simulink model "case6"  (R2024b)
settings: Solver=FixedStepAuto  StartTime=0  StopTime=1  FixedStep=1e-7  RelTol=1e-3
values from neighbouring files (symbols this model uses):
  SG_D_1_D = 0.01056    [IEEE9_case_parameters.m]    (also in case1_parameters.m; case2_parameters.m; case3_parameters.m; case4_parameters.m)
  SG_D_1_EnableSaturation = 0    [IEEE9_case_parameters.m]    (also in case1_parameters.m; case2_parameters.m; case3_parameters.m; case4_parameters.m)
  SG_D_1_f0 = 60    [IEEE9_case_parameters.m]    (also in case1_parameters.m; case2_parameters.m; case3_parameters.m; case4_parameters.m)
  SG_D_1_H = 7.5    [IEEE9_case_parameters.m]    (also in case1_parameters.m; case2_parameters.m; case3_parameters.m; case4_parameters.m)
  SG_D_1_K_A = 20    [IEEE9_case_parameters.m]    (also in case1_parameters.m; case2_parameters.m; case3_parameters.m; case4_parameters.m)
  SG_D_1_K_E = 1.000000e+1    (= 10)    [IEEE9_case_parameters.m]    (also in case1_parameters.m; case2_parameters.m; case3_parameters.m; case4_parameters.m)
  SG_D_1_K_F = 2.363    [IEEE9_case_parameters.m]    (also in case1_parameters.m; case2_parameters.m; case3_parameters.m; case4_parameters.m)
  SG_D_1_K_s = 0.5    [IEEE9_case_parameters.m]    (also in case1_parameters.m = 5; case2_parameters.m = 5; case3_parameters.m = 5; case4_parameters.m = 5)
  SG_D_1_R_a = 0.001088    [IEEE9_case_parameters.m]    (also in case1_parameters.m; case2_parameters.m; case3_parameters.m; case4_parameters.m)
  SG_D_1_S_A = 1    [IEEE9_case_parameters.m]    (also in case1_parameters.m; case2_parameters.m; case3_parameters.m; case4_parameters.m)
  SG_D_1_S_B = 0.103    [IEEE9_case_parameters.m]    (also in case1_parameters.m; case2_parameters.m; case3_parameters.m; case4_parameters.m)
  SG_D_1_S_N = 10.659857    [IEEE9_case_parameters.m]    (also in case1_parameters.m; case2_parameters.m; case3_parameters.m; case4_parameters.m)
  SG_D_1_SpeedPara = 200    [IEEE9_case_parameters.m]    (also in case1_parameters.m; case2_parameters.m; case3_parameters.m; case4_parameters.m)
  SG_D_1_T_0 = 0.720173    [IEEE9_case_parameters.m]    (also in case1_parameters.m = 0.755522; case2_parameters.m = 0.808931; case3_parameters.m = 0.869402; case4_parameters.m = 0.729316)
  SG_D_1_T_1 = 0.3    [IEEE9_case_parameters.m]    (also in case1_parameters.m; case2_parameters.m; case3_parameters.m; case4_parameters.m)
  SG_D_1_T_2 = 0.05    [IEEE9_case_parameters.m]    (also in case1_parameters.m; case2_parameters.m; case3_parameters.m; case4_parameters.m)
  SG_D_1_T_3 = 0.02    [IEEE9_case_parameters.m]    (also in case1_parameters.m; case2_parameters.m; case3_parameters.m; case4_parameters.m)
  SG_D_1_T_4 = 0.005    [IEEE9_case_parameters.m]    (also in case1_parameters.m; case2_parameters.m; case3_parameters.m; case4_parameters.m)
  SG_D_1_T_A = 0.02    [IEEE9_case_parameters.m]    (also in case1_parameters.m; case2_parameters.m; case3_parameters.m; case4_parameters.m)
  SG_D_1_T_dd = 8.000000e+0    (= 8)    [IEEE9_case_parameters.m]    (also in case1_parameters.m; case2_parameters.m; case3_parameters.m; case4_parameters.m)
  SG_D_1_T_ddd = 0.04    [IEEE9_case_parameters.m]    (also in case1_parameters.m; case2_parameters.m; case3_parameters.m; case4_parameters.m)
  SG_D_1_T_E = 0.314    [IEEE9_case_parameters.m]    (also in case1_parameters.m; case2_parameters.m; case3_parameters.m; case4_parameters.m)
  SG_D_1_T_F = 0.35    [IEEE9_case_parameters.m]    (also in case1_parameters.m; case2_parameters.m; case3_parameters.m; case4_parameters.m)
  SG_D_1_T_qd = 0.8    [IEEE9_case_parameters.m]    (also in case1_parameters.m; case2_parameters.m; case3_parameters.m; case4_parameters.m)
  SG_D_1_T_qdd = 0.02    [IEEE9_case_parameters.m]    (also in case1_parameters.m; case2_parameters.m; case3_parameters.m; case4_parameters.m)
  SG_D_1_T_speed = 0.1    [IEEE9_case_parameters.m]    (also in case1_parameters.m = 200; case2_parameters.m = 200; case3_parameters.m = 200; case4_parameters.m = 200)
  SG_D_1_T_w = 0.5    [IEEE9_case_parameters.m]    (also in case1_parameters.m; case2_parameters.m; case3_parameters.m; case4_parameters.m)
  SG_D_1_V_ref = 1.990276    [IEEE9_case_parameters.m]    (also in case1_parameters.m = 2.042296; case2_parameters.m = 2.051388; case3_parameters.m = 2.089584; case4_parameters.m = 2.01845)
  SG_D_1_w_ref = 376.991118    [IEEE9_case_parameters.m]    (also in case1_parameters.m; case2_parameters.m; case3_parameters.m; case4_parameters.m)
  SG_D_1_wb = 6.000000e+1    (= 60)    [IEEE9_case_parameters.m]    (also in case1_parameters.m; case2_parameters.m; case3_parameters.m; case4_parameters.m)
  SG_D_1_x_d = 1.9    [IEEE9_case_parameters.m]    (also in case1_parameters.m; case2_parameters.m; case3_parameters.m; case4_parameters.m)
  SG_D_1_x_dd = 0.302    [IEEE9_case_parameters.m]    (also in case1_parameters.m; case2_parameters.m; case3_parameters.m; case4_parameters.m)
  SG_D_1_x_ddd = 0.204    [IEEE9_case_parameters.m]    (also in case1_parameters.m; case2_parameters.m; case3_parameters.m; case4_parameters.m)
  SG_D_1_x_l = 0.05    [IEEE9_case_parameters.m]    (also in case1_parameters.m; case2_parameters.m; case3_parameters.m; case4_parameters.m)
  SG_D_1_x_q = 1.3    [IEEE9_case_parameters.m]    (also in case1_parameters.m; case2_parameters.m; case3_parameters.m; case4_parameters.m)
  SG_D_1_x_qd = 0.5    [IEEE9_case_parameters.m]    (also in case1_parameters.m; case2_parameters.m; case3_parameters.m; case4_parameters.m)
  SG_D_1_x_qdd = 0.3    [IEEE9_case_parameters.m]    (also in case1_parameters.m; case2_parameters.m; case3_parameters.m; case4_parameters.m)
  SG_D_2_D = 0.02    [IEEE9_case_parameters.m]    (also in case1_parameters.m; case2_parameters.m; case3_parameters.m; case4_parameters.m)
  SG_D_2_EnableSaturation = 0    [IEEE9_case_parameters.m]    (also in case1_parameters.m; case2_parameters.m; case3_parameters.m; case4_parameters.m)
  SG_D_2_f0 = 60    [IEEE9_case_parameters.m]    (also in case1_parameters.m; case2_parameters.m; case3_parameters.m; case4_parameters.m)
  SG_D_2_H = 8.000000e+0    (= 8)    [IEEE9_case_parameters.m]    (also in case1_parameters.m; case2_parameters.m; case3_parameters.m; case4_parameters.m)
  SG_D_2_K_A = 20    [IEEE9_case_parameters.m]    (also in case1_parameters.m; case2_parameters.m; case3_parameters.m; case4_parameters.m)
  SG_D_2_K_E = 1.000000e+1    (= 10)    [IEEE9_case_parameters.m]    (also in case1_parameters.m; case2_parameters.m; case3_parameters.m; case4_parameters.m)
  SG_D_2_K_F = 2.363    [IEEE9_case_parameters.m]    (also in case1_parameters.m; case2_parameters.m; case3_parameters.m; case4_parameters.m)
  SG_D_2_K_s = 0.5    [IEEE9_case_parameters.m]    (also in case1_parameters.m = 4; case2_parameters.m = 4; case3_parameters.m = 4; case4_parameters.m = 4)
  SG_D_2_R_a = 0.001088    [IEEE9_case_parameters.m]    (also in case1_parameters.m; case2_parameters.m; case3_parameters.m; case4_parameters.m)
  SG_D_2_S_A = 1    [IEEE9_case_parameters.m]    (also in case1_parameters.m; case2_parameters.m; case3_parameters.m; case4_parameters.m)
  SG_D_2_S_B = 0.103    [IEEE9_case_parameters.m]    (also in case1_parameters.m; case2_parameters.m; case3_parameters.m; case4_parameters.m)
  SG_D_2_S_N = 10.659857    [IEEE9_case_parameters.m]    (also in case1_parameters.m; case2_parameters.m; case3_parameters.m; case4_parameters.m)
  SG_D_2_SpeedPara = 200    [IEEE9_case_parameters.m]    (also in case1_parameters.m; case2_parameters.m; case3_parameters.m; case4_parameters.m)
  SG_D_2_T_0 = 1.632913    [IEEE9_case_parameters.m]    (also in case1_parameters.m = 1.632925; case2_parameters.m = 1.632915; case3_parameters.m = 1.632914; case4_parameters.m = 1.632927)
  SG_D_2_T_1 = 0.2    [IEEE9_case_parameters.m]    (also in case1_parameters.m; case2_parameters.m; case3_parameters.m; case4_parameters.m)
  SG_D_2_T_2 = 0.05    [IEEE9_case_parameters.m]    (also in case1_parameters.m; case2_parameters.m; case3_parameters.m; case4_parameters.m)
  SG_D_2_T_3 = 0.02    [IEEE9_case_parameters.m]    (also in case1_parameters.m; case2_parameters.m; case3_parameters.m; case4_parameters.m)
  SG_D_2_T_4 = 0.005    [IEEE9_case_parameters.m]    (also in case1_parameters.m; case2_parameters.m; case3_parameters.m; case4_parameters.m)
  SG_D_2_T_A = 0.02    [IEEE9_case_parameters.m]    (also in case1_parameters.m; case2_parameters.m; case3_parameters.m; case4_parameters.m)
  SG_D_2_T_dd = 7.9    [IEEE9_case_parameters.m]    (also in case1_parameters.m; case2_parameters.m; case3_parameters.m; case4_parameters.m)
  SG_D_2_T_ddd = 0.04    [IEEE9_case_parameters.m]    (also in case1_parameters.m; case2_parameters.m; case3_parameters.m; case4_parameters.m)
  SG_D_2_T_E = 0.314    [IEEE9_case_parameters.m]    (also in case1_parameters.m; case2_parameters.m; case3_parameters.m; case4_parameters.m)
  SG_D_2_T_F = 0.35    [IEEE9_case_parameters.m]    (also in case1_parameters.m; case2_parameters.m; case3_parameters.m; case4_parameters.m)
  SG_D_2_T_qd = 0.8    [IEEE9_case_parameters.m]    (also in case1_parameters.m; case2_parameters.m; case3_parameters.m; case4_parameters.m)
  SG_D_2_T_qdd = 0.015    [IEEE9_case_parameters.m]    (also in case1_parameters.m; case2_parameters.m; case3_parameters.m; case4_parameters.m)
  SG_D_2_T_speed = 0.1    [IEEE9_case_parameters.m]    (also in case1_parameters.m = 150; case2_parameters.m = 150; case3_parameters.m = 150; case4_parameters.m = 150)
  SG_D_2_T_w = 0.35    [IEEE9_case_parameters.m]    (also in case1_parameters.m; case2_parameters.m; case3_parameters.m; case4_parameters.m)
  SG_D_2_V_ref = 2.58547    [IEEE9_case_parameters.m]    (also in case1_parameters.m = 2.597896; case2_parameters.m = 2.587136; case3_parameters.m = 2.586042; case4_parameters.m = 2.599679)
  SG_D_2_w_ref = 376.991118    [IEEE9_case_parameters.m]    (also in case1_parameters.m; case2_parameters.m; case3_parameters.m; case4_parameters.m)
  SG_D_2_wb = 6.000000e+1    (= 60)    [IEEE9_case_parameters.m]    (also in case1_parameters.m; case2_parameters.m; case3_parameters.m; case4_parameters.m)
  SG_D_2_x_d = 1.8    [IEEE9_case_parameters.m]    (also in case1_parameters.m; case2_parameters.m; case3_parameters.m; case4_parameters.m)
  SG_D_2_x_dd = 0.302    [IEEE9_case_parameters.m]    (also in case1_parameters.m; case2_parameters.m; case3_parameters.m; case4_parameters.m)
  SG_D_2_x_ddd = 0.204    [IEEE9_case_parameters.m]    (also in case1_parameters.m; case2_parameters.m; case3_parameters.m; case4_parameters.m)
  SG_D_2_x_l = 0.05    [IEEE9_case_parameters.m]    (also in case1_parameters.m; case2_parameters.m; case3_parameters.m; case4_parameters.m)
  SG_D_2_x_q = 1.25    [IEEE9_case_parameters.m]    (also in case1_parameters.m; case2_parameters.m; case3_parameters.m; case4_parameters.m)
  SG_D_2_x_qd = 0.5    [IEEE9_case_parameters.m]    (also in case1_parameters.m; case2_parameters.m; case3_parameters.m; case4_parameters.m)
  SG_D_2_x_qdd = 0.3    [IEEE9_case_parameters.m]    (also in case1_parameters.m; case2_parameters.m; case3_parameters.m; case4_parameters.m)
  SG_D_3_D = 0.02    [IEEE9_case_parameters.m]    (also in case1_parameters.m; case2_parameters.m; case3_parameters.m; case4_parameters.m)
  SG_D_3_EnableSaturation = 0    [IEEE9_case_parameters.m]    (also in case1_parameters.m; case2_parameters.m; case3_parameters.m; case4_parameters.m)
  SG_D_3_f0 = 60    [IEEE9_case_parameters.m]    (also in case1_parameters.m; case2_parameters.m; case3_parameters.m; case4_parameters.m)
  SG_D_3_H = 7.7    [IEEE9_case_parameters.m]    (also in case1_parameters.m; case2_parameters.m; case3_parameters.m; case4_parameters.m)
  SG_D_3_K_A = 20    [IEEE9_case_parameters.m]    (also in case1_parameters.m; case2_parameters.m; case3_parameters.m; case4_parameters.m)
  SG_D_3_K_E = 1.000000e+1    (= 10)    [IEEE9_case_parameters.m]    (also in case1_parameters.m; case2_parameters.m; case3_parameters.m; case4_parameters.m)
  SG_D_3_K_F = 2.363    [IEEE9_case_parameters.m]    (also in case1_parameters.m; case2_parameters.m; case3_parameters.m; case4_parameters.m)
  SG_D_3_K_s = 0.2    [IEEE9_case_parameters.m]    (also in case1_parameters.m = 2; case2_parameters.m = 2; case3_parameters.m = 2; case4_parameters.m = 2)
  SG_D_3_R_a = 0.001088    [IEEE9_case_parameters.m]    (also in case1_parameters.m; case2_parameters.m; case3_parameters.m; case4_parameters.m)
  SG_D_3_S_A = 1    [IEEE9_case_parameters.m]    (also in case1_parameters.m; case2_parameters.m; case3_parameters.m; case4_parameters.m)
  SG_D_3_S_B = 0.103    [IEEE9_case_parameters.m]    (also in case1_parameters.m; case2_parameters.m; case3_parameters.m; case4_parameters.m)
  SG_D_3_S_N = 10.659857    [IEEE9_case_parameters.m]    (also in case1_parameters.m; case2_parameters.m; case3_parameters.m; case4_parameters.m)
  SG_D_3_SpeedPara = 200    [IEEE9_case_parameters.m]    (also in case1_parameters.m; case2_parameters.m; case3_parameters.m; case4_parameters.m)
  SG_D_3_T_0 = 0.850788    [IEEE9_case_parameters.m]    (also in case1_parameters.m = 0.850786; case2_parameters.m = 0.850787; case3_parameters.m; case4_parameters.m = 0.850786)
  SG_D_3_T_1 = 0.2    [IEEE9_case_parameters.m]    (also in case1_parameters.m; case2_parameters.m; case3_parameters.m; case4_parameters.m)
  SG_D_3_T_2 = 0.05    [IEEE9_case_parameters.m]    (also in case1_parameters.m; case2_parameters.m; case3_parameters.m; case4_parameters.m)
  SG_D_3_T_3 = 0.02    [IEEE9_case_parameters.m]    (also in case1_parameters.m; case2_parameters.m; case3_parameters.m; case4_parameters.m)
  SG_D_3_T_4 = 0.005    [IEEE9_case_parameters.m]    (also in case1_parameters.m; case2_parameters.m; case3_parameters.m; case4_parameters.m)
  SG_D_3_T_A = 0.02    [IEEE9_case_parameters.m]    (also in case1_parameters.m; case2_parameters.m; case3_parameters.m; case4_parameters.m)
  SG_D_3_T_dd = 8.1    [IEEE9_case_parameters.m]    (also in case1_parameters.m; case2_parameters.m; case3_parameters.m; case4_parameters.m)
  SG_D_3_T_ddd = 0.04    [IEEE9_case_parameters.m]    (also in case1_parameters.m; case2_parameters.m; case3_parameters.m; case4_parameters.m)
  SG_D_3_T_E = 0.314    [IEEE9_case_parameters.m]    (also in case1_parameters.m; case2_parameters.m; case3_parameters.m; case4_parameters.m)
  SG_D_3_T_F = 0.35    [IEEE9_case_parameters.m]    (also in case1_parameters.m; case2_parameters.m; case3_parameters.m; case4_parameters.m)
  SG_D_3_T_qd = 0.8    [IEEE9_case_parameters.m]    (also in case1_parameters.m; case2_parameters.m; case3_parameters.m; case4_parameters.m)
  SG_D_3_T_qdd = 0.015    [IEEE9_case_parameters.m]    (also in case1_parameters.m; case2_parameters.m; case3_parameters.m; case4_parameters.m)
  SG_D_3_T_speed = 0.1    [IEEE9_case_parameters.m]    (also in case1_parameters.m = 180; case2_parameters.m = 180; case3_parameters.m = 180; case4_parameters.m = 180)
  SG_D_3_T_w = 0.4    [IEEE9_case_parameters.m]    (also in case1_parameters.m; case2_parameters.m; case3_parameters.m; case4_parameters.m)
  SG_D_3_V_ref = 1.892727    [IEEE9_case_parameters.m]    (also in case1_parameters.m = 1.906439; case2_parameters.m = 1.895535; case3_parameters.m = 1.892105; case4_parameters.m = 1.906598)
  SG_D_3_w_ref = 376.991118    [IEEE9_case_parameters.m]    (also in case1_parameters.m; case2_parameters.m; case3_parameters.m; case4_parameters.m)
  SG_D_3_wb = 6.000000e+1    (= 60)    [IEEE9_case_parameters.m]    (also in case1_parameters.m; case2_parameters.m; case3_parameters.m; case4_parameters.m)
  SG_D_3_x_d = 1.85    [IEEE9_case_parameters.m]    (also in case1_parameters.m; case2_parameters.m; case3_parameters.m; case4_parameters.m)
  SG_D_3_x_dd = 0.302    [IEEE9_case_parameters.m]    (also in case1_parameters.m; case2_parameters.m; case3_parameters.m; case4_parameters.m)
  SG_D_3_x_ddd = 0.204    [IEEE9_case_parameters.m]    (also in case1_parameters.m; case2_parameters.m; case3_parameters.m; case4_parameters.m)
  SG_D_3_x_l = 0.05    [IEEE9_case_parameters.m]    (also in case1_parameters.m; case2_parameters.m; case3_parameters.m; case4_parameters.m)
  SG_D_3_x_q = 1.2    [IEEE9_case_parameters.m]    (also in case1_parameters.m; case2_parameters.m; case3_parameters.m; case4_parameters.m)
  SG_D_3_x_qd = 0.5    [IEEE9_case_parameters.m]    (also in case1_parameters.m; case2_parameters.m; case3_parameters.m; case4_parameters.m)
  SG_D_3_x_qdd = 0.3    [IEEE9_case_parameters.m]    (also in case1_parameters.m; case2_parameters.m; case3_parameters.m; case4_parameters.m)
(part 10 of 12)

== system case6/SG_D_3/d_R_f_SG_D_3_block ==
  note: d_R_f_SG_D_3 in case6
      | $-\frac{R_{f,\mathrm{SG},D,3}-\frac{E_{\mathrm{fd},\mathrm{SG},D,3}\,K_{F}}{T_{F}}}{T_{F}}$
      | Automatically generated on 2025-10-31 19:19:44 .
  State_E_fd_SG_D_3_171e0 : Inport
  State_R_f_SG_D_3_894c1 : Inport  Port=2
  Constant_K_F_19433 : Constant  Value=K_F
  Constant_T_F_4ec61 : Constant  Value=T_F
  Constant_T_F_b216c : Constant  Value=T_F
  Divide_06bee : Product  Inputs=*/
  Divide_27434 : Product  Inputs=*/
  Product_69345 : Product
  Subtract_db232 : Sum  Inputs=+-
  Blockout_d_R_f_SG_D_3_3e157 : Outport
  wires:
  State_E_fd_SG_D_3_171e0/1 -> Product_69345/1
  Constant_T_F_4ec61/1 -> Divide_27434/2
  Constant_K_F_19433/1 -> Product_69345/2
  Product_69345/1 -> Divide_27434/1
  Divide_27434/1 -> Subtract_db232/1
  State_R_f_SG_D_3_894c1/1 -> Subtract_db232/2
  Subtract_db232/1 -> Divide_06bee/1
  Constant_T_F_b216c/1 -> Divide_06bee/2
  Divide_06bee/1 -> Blockout_d_R_f_SG_D_3_3e157/1

== system case6/SG_D_3/d_T_m_SG_D_3_block ==
  note: d_T_m_SG_D_3 in case6
      | $-\frac{T_{m,\mathrm{SG},D,3}-T_{0}+\frac{\mathrm{SpeedPara}\,\left(w_{\mathrm{SG},D,3}-w_{\mathrm{ref}}\right)}{2\,f_{0}\,\pi }}{T_{\mathrm{speed}}}$
      | Automatically generated on 2025-10-31 19:19:32 .
  State_w_SG_D_3_7ff4f : Inport
  State_T_m_SG_D_3_3eb97 : Inport  Port=2
  Add_3f921 : Sum
  Add_cac69 : Sum
  Constant_-1_5abbc : Constant  Value=-1
  Constant_2.0_37fb5 : Constant  Value=2.0
  Constant_SpeedPara_197a0 : Constant  Value=SpeedPara
  Constant_T_0_e73f1 : Constant  Value=T_0
  Constant_T_speed_89bdf : Constant  Value=T_speed
  Constant_f0_63a22 : Constant  Value=f0
  Constant_pi_6d414 : Constant  Value=pi
  Constant_w_ref_18813 : Constant  Value=w_ref
  Divide_450e2 : Product  Inputs=*/
  Divide_507ef : Product  Inputs=*/
  Product_50c42 : Product
  Product_96e53 : Product
  Product_b147d : Product
  Product_ddc0b : Product
  Subtract_802e0 : Sum  Inputs=+-
  Blockout_d_T_m_SG_D_3_a2b29 : Outport
  wires:
  Constant_SpeedPara_197a0/1 -> Product_96e53/1
  Constant_-1_5abbc/1 -> Product_ddc0b/1
  Constant_w_ref_18813/1 -> Add_cac69/2
  State_w_SG_D_3_7ff4f/1 -> Product_ddc0b/2
  Constant_2.0_37fb5/1 -> Product_b147d/1
  Product_ddc0b/1 -> Add_cac69/1
  Constant_pi_6d414/1 -> Product_b147d/2
  Add_cac69/1 -> Product_96e53/2
  Product_b147d/1 -> Product_50c42/1
  Constant_f0_63a22/1 -> Product_50c42/2
  Product_96e53/1 -> Divide_450e2/1
  Product_50c42/1 -> Divide_450e2/2
  Divide_450e2/1 -> Add_3f921/1
  Constant_T_0_e73f1/1 -> Add_3f921/2
  Add_3f921/1 -> Subtract_802e0/1
  State_T_m_SG_D_3_3eb97/1 -> Subtract_802e0/2
  Subtract_802e0/1 -> Divide_507ef/1
  Constant_T_speed_89bdf/1 -> Divide_507ef/2
  Divide_507ef/1 -> Blockout_d_T_m_SG_D_3_a2b29/1

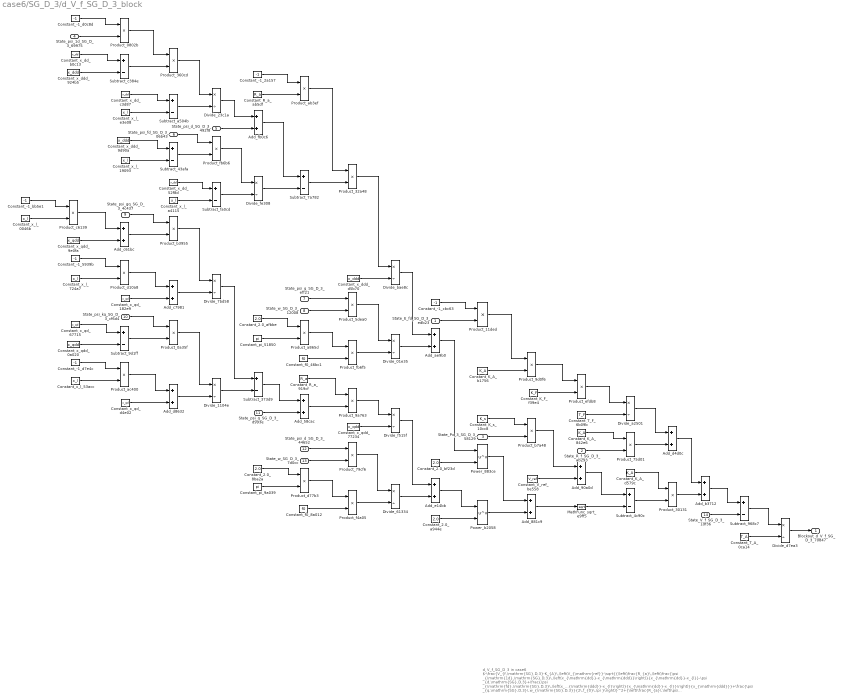
== system case6/SG_D_3/d_V_f_SG_D_3_block ==
  note: d_V_f_SG_D_3 in case6
      | $-\frac{V_{f,\mathrm{SG},D,3}-K_{A}\,\left(V_{\mathrm{ref}}-\sqrt{{\left(\frac{R_{a}\,\left(\frac{\psi _{\mathrm{1d},\mathrm{SG},D,3}\,\left(x_{\mathrm{dd}}-x_{\mathrm{ddd}}\right)}{x_{\mathrm{dd}}-x_{l}}-\psi _{d,\mathrm{SG},D,3}+\frac{\psi _{\mathrm{fd},\mathrm{SG},D,3}\,\left(x_{\mathrm{ddd}}-x_{l}\right)}{x_{\mathrm{dd}}-x_{l}}\right)}{x_{\mathrm{ddd}}}+\frac{\psi _{q,\mathrm{SG},D,3}\,w_{\mathrm{SG},D,3}}{2\,f_{0}\,\pi }\right)}^2+{\left(\frac{R_{a}\,\left(\psi _{q,\mathrm{SG},D,3}+\frac{\psi _{\mathrm{gq},\mathrm{SG},D,3}\,\left(x_{l}-x_{\mathrm{qdd}}\right)}{x_{l}-x_{\mathrm{qd}}}+\frac{\psi _{\mathrm{kq},\mathrm{SG},D,3}\,\left(x_{\mathrm{qd}}-x_{\mathrm{qdd}}\right)}{x_{l}-x_{\mathrm{qd}}}\right)}{x_{\mathrm{qdd}}}+\frac{\psi _{d,\mathrm{SG},D,3}\,w_{\mathrm{SG},D,3}}{2\,f_{0}\,\pi }\right)}^2}+K_{s}\,\mathrm{Px}_{3,\mathrm{SG},D,3}\right)-K_{A}\,R_{f,\mathrm{SG},D,3}+\frac{E_{\mathrm{fd},\mathrm{SG},D,3}\,K_{A}\,K_{F}}{T_{F}}}{T_{A}}$
      | Automatically generated on 2025-10-31 19:19:42 .
  State_E_fd_SG_D_3_edb23 : Inport
  State_R_f_SG_D_3_ab293 : Inport  Port=2
  State_Px_3_SG_D_3_58129 : Inport  Port=3
  State_psi_1d_SG_D_3_69975 : Inport  Port=4
  State_psi_d_SG_D_3_492f8 : Inport  Port=5
  State_psi_fd_SG_D_3_06b43 : Inport  Port=6
  State_psi_q_SG_D_3_eff21 : Inport  Port=7
  State_w_SG_D_3_12008 : Inport  Port=8
  State_psi_gq_SG_D_3_4c437 : Inport  Port=9
  State_psi_kq_SG_D_3_cf6d4 : Inport  Port=10
  State_psi_q_SG_D_3_d993e : Inport  Port=11
  State_psi_d_SG_D_3_44652 : Inport  Port=12
  State_w_SG_D_3_7d0cc : Inport  Port=13
  State_V_f_SG_D_3_1df36 : Inport  Port=14
  Add_58cac : Sum
  Add_881c9 : Sum
  Add_90a0d : Sum
  Add_ae9b0 : Sum
  Add_b3712 : Sum
  Add_c61bc : Sum
  Add_c7981 : Sum
  Add_d4d0c : Sum
  Add_d8632 : Sum
  Add_e14bb : Sum
  Add_fb0c6 : Sum
  Constant_-1_2a157 : Constant  Value=-1
  Constant_-1_5939b : Constant  Value=-1
  Constant_-1_bb5e1 : Constant  Value=-1
  Constant_-1_cbc63 : Constant  Value=-1
  Constant_-1_d0c8d : Constant  Value=-1
  Constant_-1_d7e4c : Constant  Value=-1
  Constant_2.0_8ba2a : Constant  Value=2.0
  Constant_2.0_a944e : Constant  Value=2.0
  Constant_2.0_afbbe : Constant  Value=2.0
  Constant_2.0_bf23d : Constant  Value=2.0
  Constant_K_A_842e6 : Constant  Value=K_A
  Constant_K_A_b1756 : Constant  Value=K_A
  Constant_K_A_d579c : Constant  Value=K_A
  Constant_K_F_f39e4 : Constant  Value=K_F
  Constant_K_s_10cc8 : Constant  Value=K_s
  Constant_R_a_919cf : Constant  Value=R_a
  Constant_R_a_ab5df : Constant  Value=R_a
  Constant_T_A_0ca14 : Constant  Value=T_A
  Constant_T_F_6b09b : Constant  Value=T_F
  Constant_V_ref_be558 : Constant  Value=V_ref
  Constant_f0_46bc1 : Constant  Value=f0
  Constant_f0_8a012 : Constant  Value=f0
  Constant_pi_51850 : Constant  Value=pi
  Constant_pi_9a039 : Constant  Value=pi
  Constant_x_dd_52f8d : Constant  Value=x_dd
  Constant_x_dd_b0c13 : Constant  Value=x_dd
  Constant_x_dd_c3d87 : Constant  Value=x_dd
  Constant_x_ddd_924b5 : Constant  Value=x_ddd
  Constant_x_ddd_9d90a : Constant  Value=x_ddd
  Constant_x_ddd_d5b70 : Constant  Value=x_ddd
  Constant_x_l_0046b : Constant  Value=x_l
  Constant_x_l_19093 : Constant  Value=x_l
  Constant_x_l_53acc : Constant  Value=x_l
  Constant_x_l_724a7 : Constant  Value=x_l
  Constant_x_l_a4115 : Constant  Value=x_l
  Constant_x_l_e3e08 : Constant  Value=x_l
  Constant_x_qd_182e9 : Constant  Value=x_qd
  Constant_x_qd_67715 : Constant  Value=x_qd
  Constant_x_qd_d4e02 : Constant  Value=x_qd
  Constant_x_qdd_0a020 : Constant  Value=x_qdd
  Constant_x_qdd_77234 : Constant  Value=x_qdd
  Constant_x_qdd_9e0fa : Constant  Value=x_qdd
  Divide_01e35 : Product  Inputs=*/
  Divide_1104e : Product  Inputs=*/
  Divide_23c1a : Product  Inputs=*/
  Divide_61334 : Product  Inputs=*/
  Divide_7bd58 : Product  Inputs=*/
  Divide_a2501 : Product  Inputs=*/
  Divide_bae8c : Product  Inputs=*/
  Divide_d7ea3 : Product  Inputs=*/
  Divide_f515f : Product  Inputs=*/
  Divide_fe308 : Product  Inputs=*/
  MathFunc_sqrt_e9ff5 : Sqrt
  Power_883ce : Math  Operator=pow
  Power_b2058 : Math  Operator=pow
  Product_0802b : Product
  Product_0a35f : Product
  Product_11ded : Product
  Product_30131 : Product
  Product_32a48 : Product
  Product_360cd : Product
  Product_5dea0 : Product
  Product_75d01 : Product
  Product_79cf6 : Product
  Product_9a763 : Product
  Product_9d0f6 : Product
  Product_a865d : Product
  Product_ab3ef : Product
  Product_ac400 : Product
  Product_b3955 : Product
  Product_b7a48 : Product
  Product_c6139 : Product
  Product_d10a8 : Product
  Product_d77b3 : Product
  Product_efdb8 : Product
  Product_f4a05 : Product
  Product_fb6b6 : Product
  Product_fb6f5 : Product
  Subtract_373d9 : Sum  Inputs=+-
  Subtract_43afa : Sum  Inputs=+-
  Subtract_4c90c : Sum  Inputs=+-
  Subtract_7a782 : Sum  Inputs=+-
  Subtract_968c7 : Sum  Inputs=+-
  Subtract_9d1ff : Sum  Inputs=+-
  Subtract_a504b : Sum  Inputs=+-
  Subtract_c384e : Sum  Inputs=+-
  Subtract_fa0cd : Sum  Inputs=+-
  Blockout_d_V_f_SG_D_3_70847 : Outport
  wires:
  Constant_K_A_842e6/1 -> Product_75d01/1
  Constant_-1_bb5e1/1 -> Product_c6139/1
  Subtract_43afa/1 -> Product_fb6b6/2
  Constant_x_l_0046b/1 -> Product_c6139/2
  Divide_61334/1 -> Add_e14bb/2
  Constant_-1_d0c8d/1 -> Product_0802b/1
  State_psi_1d_SG_D_3_69975/1 -> Product_0802b/2
  Constant_x_dd_b0c13/1 -> Subtract_c384e/1
  Divide_fe308/1 -> Subtract_7a782/2
  Product_c6139/1 -> Add_c61bc/1
  Constant_x_qdd_9e0fa/1 -> Add_c61bc/2
  Constant_x_ddd_924b5/1 -> Subtract_c384e/2
  Constant_2.0_a944e/1 -> Power_b2058/2
  Constant_-1_5939b/1 -> Product_d10a8/1
  Divide_7bd58/1 -> Subtract_373d9/1
  Subtract_a504b/1 -> Divide_23c1a/2
  Constant_x_l_724a7/1 -> Product_d10a8/2
  Constant_x_qd_67715/1 -> Subtract_9d1ff/1
  State_w_SG_D_3_12008/1 -> Product_5dea0/2
  Constant_x_qdd_0a020/1 -> Subtract_9d1ff/2
  Constant_2.0_afbbe/1 -> Product_a865d/1
  Constant_-1_d7e4c/1 -> Product_ac400/1
  Constant_pi_51850/1 -> Product_a865d/2
  Add_fb0c6/1 -> Subtract_7a782/1
  Constant_x_l_53acc/1 -> Product_ac400/2
  Product_0802b/1 -> Product_360cd/1
  Subtract_c384e/1 -> Product_360cd/2
  Constant_2.0_8ba2a/1 -> Product_d77b3/1
  Constant_x_dd_c3d87/1 -> Subtract_a504b/1
  Constant_pi_9a039/1 -> Product_d77b3/2
  Constant_x_l_e3e08/1 -> Subtract_a504b/2
  Constant_x_ddd_9d90a/1 -> Subtract_43afa/1
  Constant_x_l_19093/1 -> Subtract_43afa/2
  State_psi_gq_SG_D_3_4c437/1 -> Product_b3955/1
  Constant_x_l_a4115/1 -> Subtract_fa0cd/2
  Add_c61bc/1 -> Product_b3955/2
  Product_d10a8/1 -> Add_c7981/1
  Product_b3955/1 -> Divide_7bd58/1
  Constant_x_qd_182e9/1 -> Add_c7981/2
  State_psi_kq_SG_D_3_cf6d4/1 -> Product_0a35f/1
  State_psi_q_SG_D_3_eff21/1 -> Product_5dea0/1
  Add_ae9b0/1 -> Power_883ce/1
  Subtract_9d1ff/1 -> Product_0a35f/2
  Constant_f0_46bc1/1 -> Product_fb6f5/2
  Product_a865d/1 -> Product_fb6f5/1
  Constant_x_qd_d4e02/1 -> Add_d8632/2
  Product_ac400/1 -> Add_d8632/1
  Product_360cd/1 -> Divide_23c1a/1
  State_psi_fd_SG_D_3_06b43/1 -> Product_fb6b6/1
  Constant_x_dd_52f8d/1 -> Subtract_fa0cd/1
  Add_c7981/1 -> Divide_7bd58/2
  Add_881c9/1 -> MathFunc_sqrt_e9ff5/1
  Product_0a35f/1 -> Divide_1104e/1
  Add_d8632/1 -> Divide_1104e/2
  Product_ab3ef/1 -> Product_32a48/1
  Divide_23c1a/1 -> Add_fb0c6/1
  Add_90a0d/1 -> Subtract_4c90c/1
  State_psi_d_SG_D_3_492f8/1 -> Add_fb0c6/2
  Product_fb6b6/1 -> Divide_fe308/1
  Subtract_fa0cd/1 -> Divide_fe308/2
  MathFunc_sqrt_e9ff5/1 -> Subtract_4c90c/2
  Divide_1104e/1 -> Subtract_373d9/2
  Constant_-1_2a157/1 -> Product_ab3ef/1
  Constant_R_a_ab5df/1 -> Product_ab3ef/2
  Subtract_373d9/1 -> Add_58cac/1
  State_psi_q_SG_D_3_d993e/1 -> Add_58cac/2
  Subtract_7a782/1 -> Product_32a48/2
  Constant_R_a_919cf/1 -> Product_9a763/1
  Add_58cac/1 -> Product_9a763/2
  State_psi_d_SG_D_3_44652/1 -> Product_79cf6/1
  State_w_SG_D_3_7d0cc/1 -> Product_79cf6/2
  Product_d77b3/1 -> Product_f4a05/1
  Constant_f0_8a012/1 -> Product_f4a05/2
  Product_32a48/1 -> Divide_bae8c/1
  Constant_x_ddd_d5b70/1 -> Divide_bae8c/2
  Product_5dea0/1 -> Divide_01e35/1
  Product_fb6f5/1 -> Divide_01e35/2
  Product_9a763/1 -> Divide_f515f/1
  Constant_x_qdd_77234/1 -> Divide_f515f/2
  Product_79cf6/1 -> Divide_61334/1
  Product_f4a05/1 -> Divide_61334/2
  Divide_bae8c/1 -> Add_ae9b0/1
  Divide_01e35/1 -> Add_ae9b0/2
  Divide_f515f/1 -> Add_e14bb/1
  Constant_-1_cbc63/1 -> Product_11ded/1
  State_E_fd_SG_D_3_edb23/1 -> Product_11ded/2
  Constant_2.0_bf23d/1 -> Power_883ce/2
  Add_e14bb/1 -> Power_b2058/1
  Product_11ded/1 -> Product_9d0f6/1
  Constant_K_A_b1756/1 -> Product_9d0f6/2
  Constant_K_s_10cc8/1 -> Product_b7a48/1
  State_Px_3_SG_D_3_58129/1 -> Product_b7a48/2
  Power_883ce/1 -> Add_881c9/1
  Power_b2058/1 -> Add_881c9/2
  Product_9d0f6/1 -> Product_efdb8/1
  Constant_K_F_f39e4/1 -> Product_efdb8/2
  Product_b7a48/1 -> Add_90a0d/1
  Constant_V_ref_be558/1 -> Add_90a0d/2
  Product_efdb8/1 -> Divide_a2501/1
  Constant_T_F_6b09b/1 -> Divide_a2501/2
  Add_b3712/1 -> Subtract_968c7/1
  State_R_f_SG_D_3_ab293/1 -> Product_75d01/2
  Divide_a2501/1 -> Add_d4d0c/1
  Product_75d01/1 -> Add_d4d0c/2
  Constant_K_A_d579c/1 -> Product_30131/1
  Subtract_4c90c/1 -> Product_30131/2
  Add_d4d0c/1 -> Add_b3712/1
  Product_30131/1 -> Add_b3712/2
  State_V_f_SG_D_3_1df36/1 -> Subtract_968c7/2
  Subtract_968c7/1 -> Divide_d7ea3/1
  Constant_T_A_0ca14/1 -> Divide_d7ea3/2
  Divide_d7ea3/1 -> Blockout_d_V_f_SG_D_3_70847/1

== system case6/SG_D_3/d_psi_1d_SG_D_3_block ==
  note: d_psi_1d_SG_D_3 in case6
      | $-\frac{\psi _{\mathrm{1d},\mathrm{SG},D,3}-\psi _{\mathrm{fd},\mathrm{SG},D,3}+\frac{\left(x_{\mathrm{dd}}-x_{l}\right)\,\left(\frac{\psi _{\mathrm{1d},\mathrm{SG},D,3}\,\left(x_{\mathrm{dd}}-x_{\mathrm{ddd}}\right)}{x_{\mathrm{dd}}-x_{l}}-\psi _{d,\mathrm{SG},D,3}+\frac{\psi _{\mathrm{fd},\mathrm{SG},D,3}\,\left(x_{\mathrm{ddd}}-x_{l}\right)}{x_{\mathrm{dd}}-x_{l}}\right)}{x_{\mathrm{ddd}}}}{T_{\mathrm{ddd}}}$
      | Automatically generated on 2025-10-31 19:19:10 .
  State_psi_1d_SG_D_3_8c5b0 : Inport
  State_psi_fd_SG_D_3_60e66 : Inport  Port=2
  State_psi_1d_SG_D_3_8d87a : Inport  Port=3
  State_psi_d_SG_D_3_b075c : Inport  Port=4
  State_psi_fd_SG_D_3_e1029 : Inport  Port=5
  Add_05b45 : Sum
  Add_05c65 : Sum
  Add_32d0c : Sum
  Constant_-1_63cbd : Constant  Value=-1
  Constant_-1_fcb6e : Constant  Value=-1
  Constant_T_ddd_86f72 : Constant  Value=T_ddd
  Constant_x_dd_52070 : Constant  Value=x_dd
  Constant_x_dd_7c037 : Constant  Value=x_dd
  Constant_x_dd_e8732 : Constant  Value=x_dd
  Constant_x_dd_f259d : Constant  Value=x_dd
  Constant_x_ddd_2e5f7 : Constant  Value=x_ddd
  Constant_x_ddd_7f53f : Constant  Value=x_ddd
  Constant_x_ddd_f8590 : Constant  Value=x_ddd
  Constant_x_l_7eda9 : Constant  Value=x_l
  Constant_x_l_92282 : Constant  Value=x_l
  Constant_x_l_ad56a : Constant  Value=x_l
  Constant_x_l_c4377 : Constant  Value=x_l
  Divide_16eeb : Product  Inputs=*/
  Divide_27216 : Product  Inputs=*/
  Divide_8b2cb : Product  Inputs=*/
  Divide_d00b9 : Product  Inputs=*/
  Product_0225a : Product
  Product_2f584 : Product
  Product_8316d : Product
  Product_9e153 : Product
  Product_e1326 : Product
  Subtract_28795 : Sum  Inputs=+-
  Subtract_ade78 : Sum  Inputs=+-
  Subtract_b148d : Sum  Inputs=+-
  Subtract_cec1d : Sum  Inputs=+-
  Subtract_dd71a : Sum  Inputs=+-
  Subtract_f7884 : Sum  Inputs=+-
  Blockout_d_psi_1d_SG_D_3_f8e09 : Outport
  wires:
  Divide_27216/1 -> Add_05c65/1
  Subtract_dd71a/1 -> Product_0225a/2
  Constant_-1_fcb6e/1 -> Product_2f584/1
  Constant_x_dd_7c037/1 -> Subtract_b148d/1
  State_psi_1d_SG_D_3_8d87a/1 -> Product_2f584/2
  Product_2f584/1 -> Product_0225a/1
  Constant_x_dd_52070/1 -> Subtract_dd71a/1
  Constant_x_ddd_2e5f7/1 -> Subtract_dd71a/2
  Constant_x_l_ad56a/1 -> Subtract_b148d/2
  Constant_x_ddd_7f53f/1 -> Subtract_ade78/1
  Divide_d00b9/1 -> Blockout_d_psi_1d_SG_D_3_f8e09/1
  Constant_x_l_92282/1 -> Subtract_ade78/2
  Product_0225a/1 -> Divide_27216/1
  Subtract_b148d/1 -> Divide_27216/2
  State_psi_fd_SG_D_3_e1029/1 -> Product_8316d/1
  Subtract_ade78/1 -> Product_8316d/2
  Constant_x_dd_e8732/1 -> Subtract_28795/1
  Constant_x_l_c4377/1 -> Subtract_28795/2
  State_psi_d_SG_D_3_b075c/1 -> Add_05c65/2
  Product_8316d/1 -> Divide_8b2cb/1
  Subtract_28795/1 -> Divide_8b2cb/2
  Constant_x_dd_f259d/1 -> Subtract_f7884/1
  Constant_x_l_7eda9/1 -> Subtract_f7884/2
  Add_05c65/1 -> Subtract_cec1d/1
  Divide_8b2cb/1 -> Subtract_cec1d/2
  Constant_-1_63cbd/1 -> Product_e1326/1
  State_psi_1d_SG_D_3_8c5b0/1 -> Product_e1326/2
  State_psi_fd_SG_D_3_60e66/1 -> Add_32d0c/2
  Subtract_f7884/1 -> Product_9e153/1
  Subtract_cec1d/1 -> Product_9e153/2
  Product_e1326/1 -> Add_32d0c/1
  Product_9e153/1 -> Divide_16eeb/1
  Constant_x_ddd_f8590/1 -> Divide_16eeb/2
  Add_32d0c/1 -> Add_05b45/1
  Divide_16eeb/1 -> Add_05b45/2
  Add_05b45/1 -> Divide_d00b9/1
  Constant_T_ddd_86f72/1 -> Divide_d00b9/2

== system case6/SG_D_3/d_psi_d_SG_D_3_block ==
  note: d_psi_d_SG_D_3 in case6
      | $2\,\pi \,f_{0}\,\left(v_{d,\mathrm{SG},D,3}\,\sin\left(\theta _{\mathrm{SG},D,3}\right)-v_{q,\mathrm{SG},D,3}\,\cos\left(\theta _{\mathrm{SG},D,3}\right)+\frac{R_{a}\,\left(\frac{\psi _{\mathrm{1d},\mathrm{SG},D,3}\,\left(x_{\mathrm{dd}}-x_{\mathrm{ddd}}\right)}{x_{\mathrm{dd}}-x_{l}}-\psi _{d,\mathrm{SG},D,3}+\frac{\psi _{\mathrm{fd},\mathrm{SG},D,3}\,\left(x_{\mathrm{ddd}}-x_{l}\right)}{x_{\mathrm{dd}}-x_{l}}\right)}{x_{\mathrm{ddd}}}+\frac{\psi _{q,\mathrm{SG},D,3}\,w_{\mathrm{SG},D,3}}{2\,f_{0}\,\pi }\right)$
      | Automatically generated on 2025-10-31 19:18:54 .
  State_psi_1d_SG_D_3_bf921 : Inport
  State_psi_d_SG_D_3_ef1bf : Inport  Port=2
  State_psi_fd_SG_D_3_948b2 : Inport  Port=3
  Input_v_d_SG_D_3_f4246 : Inport  Port=4
  State_theta_SG_D_3_420f3 : Inport  Port=5
  Input_v_q_SG_D_3_8b8d5 : Inport  Port=6
  State_theta_SG_D_3_6650a : Inport  Port=7
  State_psi_q_SG_D_3_688d6 : Inport  Port=8
  State_w_SG_D_3_524fa : Inport  Port=9
  Add_1a87c : Sum
  Add_ee316 : Sum
  Constant_-1_fd2f4 : Constant  Value=-1
  Constant_-2.0_de471 : Constant  Value=-2.0
  Constant_2.0_828ac : Constant  Value=2.0
  Constant_R_a_9cb2b : Constant  Value=R_a
  Constant_f0_a7b9c : Constant  Value=f0
  Constant_f0_e9d35 : Constant  Value=f0
  Constant_pi_2d9a2 : Constant  Value=pi
  Constant_pi_a0b40 : Constant  Value=pi
  Constant_x_dd_221ec : Constant  Value=x_dd
  Constant_x_dd_38f81 : Constant  Value=x_dd
  Constant_x_dd_c8e00 : Constant  Value=x_dd
  Constant_x_ddd_5c586 : Constant  Value=x_ddd
  Constant_x_ddd_7c992 : Constant  Value=x_ddd
  Constant_x_ddd_d388d : Constant  Value=x_ddd
  Constant_x_l_7fc11 : Constant  Value=x_l
  Constant_x_l_93bf7 : Constant  Value=x_l
  Constant_x_l_a4e68 : Constant  Value=x_l
  Divide_287e3 : Product  Inputs=*/
  Divide_48070 : Product  Inputs=*/
  Divide_c61c2 : Product  Inputs=*/
  Divide_f564d : Product  Inputs=*/
  MathFunc_cos_ad870 : Trigonometry  Operator=cos
  MathFunc_sin_c140c : Trigonometry
  Product_2b40e : Product
  Product_37437 : Product
  Product_3c159 : Product
  Product_3e4d2 : Product
  Product_53a1a : Product
  Product_6997e : Product
  Product_7c3aa : Product
  Product_7d6e4 : Product
  Product_90d85 : Product
  Product_ba7f6 : Product
  Product_d1f79 : Product
  Product_d94f4 : Product
  Subtract_09268 : Sum  Inputs=+-
  Subtract_2ccb2 : Sum  Inputs=+-
  Subtract_36265 : Sum  Inputs=+-
  Subtract_403d0 : Sum  Inputs=+-
  Subtract_628c2 : Sum  Inputs=+-
  Subtract_6c74c : Sum  Inputs=+-
  Subtract_d371b : Sum  Inputs=+-
  Blockout_d_psi_d_SG_D_3_19103 : Outport
  wires:
  Constant_-1_fd2f4/1 -> Product_3c159/1
  Constant_2.0_828ac/1 -> Product_3e4d2/1
  Constant_x_dd_221ec/1 -> Subtract_09268/1
  State_psi_1d_SG_D_3_bf921/1 -> Product_3c159/2
  Constant_x_dd_38f81/1 -> Subtract_36265/1
  Constant_pi_2d9a2/1 -> Product_3e4d2/2
  Constant_x_ddd_d388d/1 -> Subtract_09268/2
  Product_3c159/1 -> Product_6997e/1
  Product_3e4d2/1 -> Product_2b40e/1
  Subtract_09268/1 -> Product_6997e/2
  Constant_-2.0_de471/1 -> Product_53a1a/1
  Constant_x_l_7fc11/1 -> Subtract_36265/2
  Constant_x_ddd_5c586/1 -> Subtract_6c74c/1
  Constant_pi_a0b40/1 -> Product_53a1a/2
  Constant_x_l_93bf7/1 -> Subtract_6c74c/2
  Product_7c3aa/1 -> Divide_287e3/1
  Product_6997e/1 -> Divide_c61c2/1
  Subtract_36265/1 -> Divide_c61c2/2
  State_psi_fd_SG_D_3_948b2/1 -> Product_37437/1
  Subtract_6c74c/1 -> Product_37437/2
  Constant_x_dd_c8e00/1 -> Subtract_403d0/1
  Constant_x_l_a4e68/1 -> Subtract_403d0/2
  Divide_287e3/1 -> Subtract_d371b/2
  Divide_c61c2/1 -> Add_ee316/1
  Subtract_628c2/1 -> Product_ba7f6/2
  State_psi_d_SG_D_3_ef1bf/1 -> Add_ee316/2
  Product_37437/1 -> Divide_f564d/1
  Subtract_403d0/1 -> Divide_f564d/2
  Add_ee316/1 -> Subtract_628c2/1
  Divide_f564d/1 -> Subtract_628c2/2
  Product_d94f4/1 -> Add_1a87c/2
  Constant_R_a_9cb2b/1 -> Product_ba7f6/1
  Product_7d6e4/1 -> Product_d1f79/1
  State_theta_SG_D_3_420f3/1 -> MathFunc_sin_c140c/1
  Product_ba7f6/1 -> Divide_48070/1
  Constant_x_ddd_7c992/1 -> Divide_48070/2
  Input_v_d_SG_D_3_f4246/1 -> Product_90d85/1
  State_w_SG_D_3_524fa/1 -> Product_7c3aa/2
  MathFunc_sin_c140c/1 -> Product_90d85/2
  State_theta_SG_D_3_6650a/1 -> MathFunc_cos_ad870/1
  MathFunc_cos_ad870/1 -> Product_d94f4/2
  Divide_48070/1 -> Subtract_2ccb2/1
  Product_90d85/1 -> Subtract_2ccb2/2
  Input_v_q_SG_D_3_8b8d5/1 -> Product_d94f4/1
  State_psi_q_SG_D_3_688d6/1 -> Product_7c3aa/1
  Constant_f0_e9d35/1 -> Product_2b40e/2
  Subtract_2ccb2/1 -> Add_1a87c/1
  Product_2b40e/1 -> Divide_287e3/2
  Product_53a1a/1 -> Product_7d6e4/1
  Constant_f0_a7b9c/1 -> Product_7d6e4/2
  Add_1a87c/1 -> Subtract_d371b/1
  Subtract_d371b/1 -> Product_d1f79/2
  Product_d1f79/1 -> Blockout_d_psi_d_SG_D_3_19103/1

== system case6/SG_D_3/d_psi_fd_SG_D_3_block ==
  note: d_psi_fd_SG_D_3 in case6
      | $-\frac{\psi _{\mathrm{fd},\mathrm{SG},D,3}-E_{\mathrm{fd},\mathrm{SG},D,3}+\left(x_{d}-x_{\mathrm{dd}}\right)\,\left(\frac{\frac{\psi _{\mathrm{1d},\mathrm{SG},D,3}\,\left(x_{\mathrm{dd}}-x_{\mathrm{ddd}}\right)}{x_{\mathrm{dd}}-x_{l}}-\psi _{d,\mathrm{SG},D,3}+\frac{\psi _{\mathrm{fd},\mathrm{SG},D,3}\,\left(x_{\mathrm{ddd}}-x_{l}\right)}{x_{\mathrm{dd}}-x_{l}}}{x_{\mathrm{ddd}}}-\frac{\left(x_{\mathrm{dd}}-x_{\mathrm{ddd}}\right)\,\left(\psi _{\mathrm{1d},\mathrm{SG},D,3}-\psi _{\mathrm{fd},\mathrm{SG},D,3}+\frac{\left(x_{\mathrm{dd}}-x_{l}\right)\,\left(\frac{\psi _{\mathrm{1d},\mathrm{SG},D,3}\,\left(x_{\mathrm{dd}}-x_{\mathrm{ddd}}\right)}{x_{\mathrm{dd}}-x_{l}}-\psi _{d,\mathrm{SG},D,3}+\frac{\psi _{\mathrm{fd},\mathrm{SG},D,3}\,\left(x_{\mathrm{ddd}}-x_{l}\right)}{x_{\mathrm{dd}}-x_{l}}\right)}{x_{\mathrm{ddd}}}\right)}{{\left(x_{\mathrm{dd}}-x_{l}\right)}^2}\right)}{T_{\mathrm{dd}}}$
      | Automatically generated on 2025-10-31 19:19:06 .
  State_E_fd_SG_D_3_340a0 : Inport
  State_psi_fd_SG_D_3_bb77c : Inport  Port=2
  State_psi_1d_SG_D_3_acd54 : Inport  Port=3
  State_psi_fd_SG_D_3_e6b96 : Inport  Port=4
  State_psi_1d_SG_D_3_a7b03 : Inport  Port=5
  State_psi_d_SG_D_3_c1f6f : Inport  Port=6
  State_psi_fd_SG_D_3_c3c1b : Inport  Port=7
  State_psi_1d_SG_D_3_8d0f1 : Inport  Port=8
  State_psi_d_SG_D_3_aa4bd : Inport  Port=9
  State_psi_fd_SG_D_3_adc17 : Inport  Port=10
  Add_3f8f2 : Sum
  Add_e415a : Sum
  Constant_-1_5fb5b : Constant  Value=-1
  Constant_-1_65cae : Constant  Value=-1
  Constant_-1_bf7ed : Constant  Value=-1
  Constant_2.0_b3d09 : Constant  Value=2.0
  Constant_T_dd_1cb39 : Constant  Value=T_dd
  Constant_x_d_39650 : Constant  Value=x_d
  Constant_x_dd_0f6c2 : Constant  Value=x_dd
  Constant_x_dd_209e9 : Constant  Value=x_dd
  Constant_x_dd_59d9d : Constant  Value=x_dd
  Constant_x_dd_77d0f : Constant  Value=x_dd
  Constant_x_dd_79a6c : Constant  Value=x_dd
  Constant_x_dd_821dd : Constant  Value=x_dd
  Constant_x_dd_9e9ed : Constant  Value=x_dd
  Constant_x_dd_a97a1 : Constant  Value=x_dd
  Constant_x_dd_c30db : Constant  Value=x_dd
  Constant_x_dd_e4a04 : Constant  Value=x_dd
  Constant_x_ddd_2bf04 : Constant  Value=x_ddd
  Constant_x_ddd_4bbae : Constant  Value=x_ddd
  Constant_x_ddd_5e6fc : Constant  Value=x_ddd
  Constant_x_ddd_788b6 : Constant  Value=x_ddd
  Constant_x_ddd_83091 : Constant  Value=x_ddd
  Constant_x_ddd_98d03 : Constant  Value=x_ddd
  Constant_x_ddd_a18d3 : Constant  Value=x_ddd
  Constant_x_l_28447 : Constant  Value=x_l
  Constant_x_l_4d2f5 : Constant  Value=x_l
  Constant_x_l_91d37 : Constant  Value=x_l
  Constant_x_l_b16bc : Constant  Value=x_l
  Constant_x_l_ce8ce : Constant  Value=x_l
  Constant_x_l_d0a56 : Constant  Value=x_l
  Constant_x_l_d2ad8 : Constant  Value=x_l
  Constant_x_l_d8ea5 : Constant  Value=x_l
  Divide_1c2c6 : Product  Inputs=*/
  Divide_4185d : Product  Inputs=*/
  Divide_5827f : Product  Inputs=*/
  Divide_5c6ba : Product  Inputs=*/
  Divide_63f54 : Product  Inputs=*/
  Divide_84caf : Product  Inputs=*/
  Divide_88a11 : Product  Inputs=*/
  Divide_b5f87 : Product  Inputs=*/
  Power_0ed8c : Math  Operator=pow
  Product_0797f : Product
  Product_2d1c7 : Product
  Product_6ce72 : Product
  Product_73a58 : Product
  Product_78b87 : Product
  Product_94222 : Product
  Product_ab23e : Product
  Product_c7994 : Product
  Product_e1ea0 : Product
  Product_f7aa0 : Product
  Subtract_10015 : Sum  Inputs=+-
  Subtract_21e2f : Sum  Inputs=+-
  Subtract_3f505 : Sum  Inputs=+-
  Subtract_6e44a : Sum  Inputs=+-
  Subtract_84296 : Sum  Inputs=+-
  Subtract_87760 : Sum  Inputs=+-
  Subtract_9949a : Sum  Inputs=+-
  Subtract_a5d57 : Sum  Inputs=+-
  Subtract_ab8bd : Sum  Inputs=+-
  Subtract_b6b84 : Sum  Inputs=+-
  Subtract_c3ff1 : Sum  Inputs=+-
  Subtract_cf681 : Sum  Inputs=+-
  Subtract_d2677 : Sum  Inputs=+-
  Subtract_d9c92 : Sum  Inputs=+-
  Subtract_dd5e5 : Sum  Inputs=+-
  Subtract_ebf48 : Sum  Inputs=+-
  Subtract_f1c3c : Sum  Inputs=+-
  Subtract_fcfe0 : Sum  Inputs=+-
  Subtract_fd2c5 : Sum  Inputs=+-
  Blockout_d_psi_fd_SG_D_3_d3b7a : Outport
  wires:
  Product_94222/1 -> Divide_b5f87/1
  Constant_-1_bf7ed/1 -> Product_f7aa0/1
  Subtract_ebf48/1 -> Product_ab23e/2
  State_psi_1d_SG_D_3_a7b03/1 -> Product_f7aa0/2
  Constant_x_l_4d2f5/1 -> Subtract_dd5e5/2
  Constant_x_dd_e4a04/1 -> Subtract_ebf48/1
  Constant_x_ddd_98d03/1 -> Subtract_ebf48/2
  Product_f7aa0/1 -> Product_ab23e/1
  Constant_x_dd_9e9ed/1 -> Subtract_a5d57/1
  Constant_x_l_d0a56/1 -> Subtract_a5d57/2
  Constant_x_ddd_788b6/1 -> Subtract_10015/2
  Constant_x_ddd_a18d3/1 -> Subtract_fd2c5/1
  Constant_x_l_b16bc/1 -> Subtract_fd2c5/2
  Product_c7994/1 -> Product_0797f/1
  Product_ab23e/1 -> Divide_88a11/1
  Subtract_a5d57/1 -> Divide_88a11/2
  State_psi_fd_SG_D_3_c3c1b/1 -> Product_6ce72/1
  Constant_x_ddd_5e6fc/1 -> Subtract_dd5e5/1
  Subtract_fd2c5/1 -> Product_6ce72/2
  Constant_x_dd_0f6c2/1 -> Subtract_c3ff1/1
  Constant_-1_5fb5b/1 -> Product_c7994/1
  Constant_x_l_d8ea5/1 -> Subtract_c3ff1/2
  Product_0797f/1 -> Divide_5827f/1
  Divide_88a11/1 -> Add_3f8f2/1
  Product_73a58/1 -> Divide_4185d/1
  State_psi_d_SG_D_3_c1f6f/1 -> Add_3f8f2/2
  State_psi_fd_SG_D_3_adc17/1 -> Product_73a58/1
  Product_6ce72/1 -> Divide_84caf/1
  Constant_x_dd_209e9/1 -> Subtract_84296/1
  Subtract_c3ff1/1 -> Divide_84caf/2
  Constant_x_l_28447/1 -> Subtract_cf681/2
  Constant_x_dd_a97a1/1 -> Subtract_ab8bd/1
  Subtract_fcfe0/1 -> Product_78b87/2
  Constant_x_l_d2ad8/1 -> Subtract_ab8bd/2
  Divide_5827f/1 -> Add_e415a/1
  Constant_x_ddd_83091/1 -> Divide_b5f87/2
  Add_3f8f2/1 -> Subtract_21e2f/1
  Divide_84caf/1 -> Subtract_21e2f/2
  State_psi_1d_SG_D_3_8d0f1/1 -> Product_c7994/2
  Constant_x_l_91d37/1 -> Subtract_84296/2
  Constant_x_dd_79a6c/1 -> Subtract_10015/1
  Subtract_ab8bd/1 -> Product_94222/1
  Add_e415a/1 -> Subtract_6e44a/1
  Subtract_21e2f/1 -> Product_94222/2
  Subtract_10015/1 -> Product_0797f/2
  Constant_x_dd_821dd/1 -> Subtract_d9c92/1
  Constant_x_l_ce8ce/1 -> Subtract_d9c92/2
  Subtract_dd5e5/1 -> Product_73a58/2
  Constant_x_dd_c30db/1 -> Subtract_fcfe0/1
  Constant_x_ddd_4bbae/1 -> Subtract_fcfe0/2
  Product_78b87/1 -> Product_e1ea0/1
  State_psi_1d_SG_D_3_acd54/1 -> Subtract_d2677/1
  Subtract_d9c92/1 -> Divide_5827f/2
  State_psi_fd_SG_D_3_e6b96/1 -> Subtract_d2677/2
  Constant_-1_65cae/1 -> Product_78b87/1
  Subtract_d2677/1 -> Subtract_3f505/1
  Divide_b5f87/1 -> Subtract_3f505/2
  Constant_x_dd_59d9d/1 -> Subtract_cf681/1
  Divide_4185d/1 -> Subtract_6e44a/2
  State_psi_d_SG_D_3_aa4bd/1 -> Add_e415a/2
  Subtract_84296/1 -> Divide_4185d/2
  Subtract_3f505/1 -> Product_e1ea0/2
  Subtract_cf681/1 -> Power_0ed8c/1
  Constant_2.0_b3d09/1 -> Power_0ed8c/2
  Product_e1ea0/1 -> Divide_63f54/1
  Subtract_87760/1 -> Product_2d1c7/2
  Power_0ed8c/1 -> Divide_63f54/2
  Subtract_6e44a/1 -> Divide_5c6ba/1
  Constant_x_ddd_2bf04/1 -> Divide_5c6ba/2
  Constant_x_d_39650/1 -> Subtract_9949a/1
  Constant_x_dd_77d0f/1 -> Subtract_9949a/2
  Divide_63f54/1 -> Subtract_87760/1
  Divide_5c6ba/1 -> Subtract_87760/2
  State_E_fd_SG_D_3_340a0/1 -> Subtract_f1c3c/1
  State_psi_fd_SG_D_3_bb77c/1 -> Subtract_f1c3c/2
  Subtract_9949a/1 -> Product_2d1c7/1
  Subtract_f1c3c/1 -> Subtract_b6b84/1
  Product_2d1c7/1 -> Subtract_b6b84/2
  Subtract_b6b84/1 -> Divide_1c2c6/1
  Constant_T_dd_1cb39/1 -> Divide_1c2c6/2
  Divide_1c2c6/1 -> Blockout_d_psi_fd_SG_D_3_d3b7a/1
